simulink library "FlatSatSelection_lib"  (R2018b)
settings: Solver=VariableStepAuto  StartTime=0.0  StopTime=10.0  RelTol=1e-3
undefined symbols (not defined in the file or in its folder): simParams
settings Model: Creator=aact_  LastModifiedBy=aact_

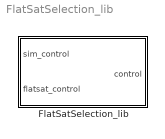
== system FlatSatSelection_lib ==
  FlatSatSelection_lib : Subsystem

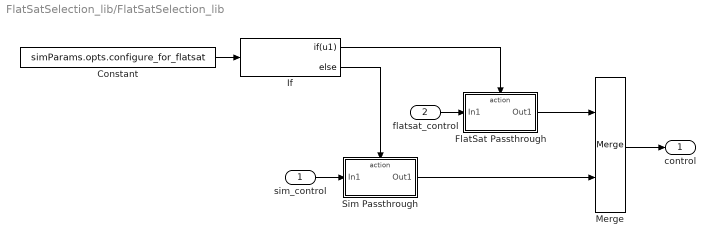
== system FlatSatSelection_lib/FlatSatSelection_lib ==
  sim_control : Inport  OutDataTypeStr=Bus: actuator_control
  flatsat_control : Inport  Port=2  OutDataTypeStr=Bus: actuator_control
  Constant : Constant  Value=simParams.opts.configure_for_flatsat
  FlatSat Passthrough : Subsystem  TreatAsAtomicUnit=on
  If : If  IfExpression=u1
  Merge : Merge
  Sim Passthrough : Subsystem  TreatAsAtomicUnit=on
  control : Outport  OutDataTypeStr=Bus: actuator_control
  wires:
  Constant/1 -> If/1
  Merge/1 -> control/1
  If/1 -> FlatSat Passthrough/Action
  FlatSat Passthrough/1(Out1) -> Merge/1
  If/2 -> Sim Passthrough/Action
  sim_control/1 -> Sim Passthrough/1(In1)
  flatsat_control/1 -> FlatSat Passthrough/1(In1)
  Sim Passthrough/1(Out1) -> Merge/2

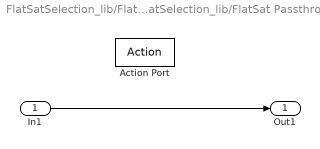
== system FlatSatSelection_lib/FlatSatSelection_lib/FlatSat Passthrough ==
  In1 : Inport
  Action Port : ActionPort  ActionType=then
  Out1 : Outport
  wires:
  In1/1 -> Out1/1

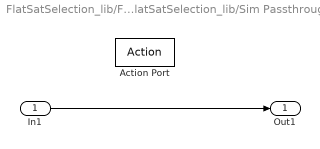
== system FlatSatSelection_lib/FlatSatSelection_lib/Sim Passthrough ==
  In1 : Inport
  Action Port : ActionPort  ActionType=else
  Out1 : Outport
  wires:
  In1/1 -> Out1/1
